simulink model "plantmodelwithcontroller"  (R2020a)
settings: Solver=VariableStepAuto  StartTime=0.0  StopTime=100  RelTol=1e-3
undefined symbols (not defined in the file): Ax, Ay, Az, b, d, g, I, Ixx, Iyy, Izz, Jr, m
libraries: simulink x4
settings Model: Creator=Muni Kumar  LastModifiedBy=Muni Kumar

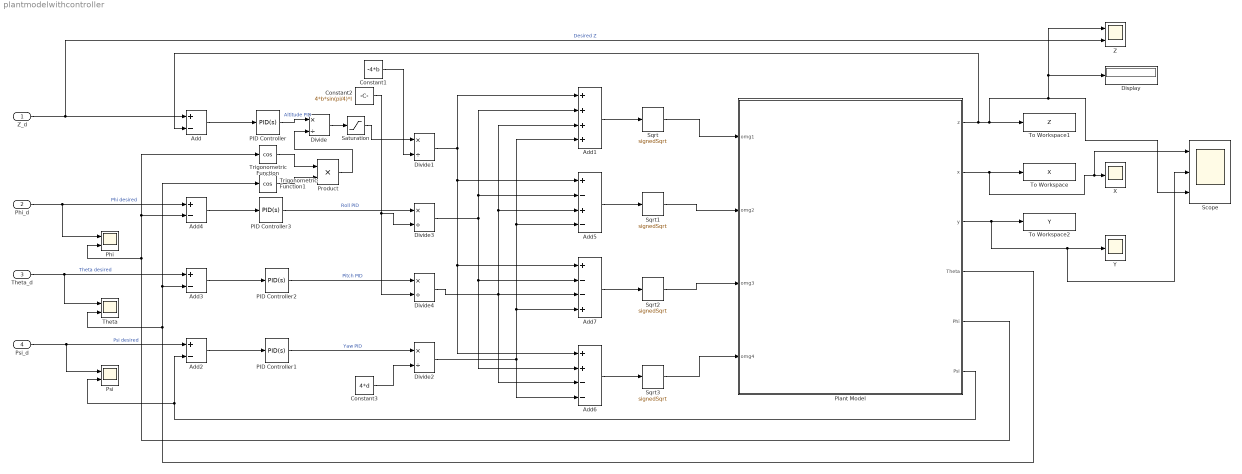
== system plantmodelwithcontroller ==
  Z_d : Inport
  Phi_d : Inport  Port=2
  Theta_d : Inport  Port=3
  Psi_d : Inport  Port=4
  Add{,2..4} (4 alike) : Sum  Inputs=+-
  Add1 : Sum  Inputs=++++
  Add5 : Sum  Inputs=+-+-
  Add6 : Sum  Inputs=++--
  Add7 : Sum  Inputs=+--+
  Constant1 : Constant  Value=-4*b
  Constant2 : Constant  Value=4*b*sin(pi/4)*I
  Constant3 : Constant  Value=4*d
  Display : Display
      settings: Decimation=2
  Divide{,1..4} (5 alike) : Product  Inputs=*/
  PID Controller : simulink/Continuous/PID Controller  Controller=PID  Form=Parallel  TimeDomain=Continuous-time  UseExternalTs=off  SampleTime=-1  IntegratorMethod=Forward Euler  FilterMethod=Forward Euler  ControllerParametersSource=internal  P=4  I=0  D=0  UseFilter=on  N=100  TunerSelectOption=Transfer Function Based (PID Tuner App)  InitialConditionSource=internal  InitialConditionForIntegrator=0  InitialConditionForFilter=0  DifferentiatorICPrevScaledInput=0  ExternalReset=none  TrackingMode=off  Kt=1  LimitOutput=off  UpperSaturationLimit=inf  LowerSaturationLimit=-inf  LinearizeAsGain=on  AntiWindupMode=none  Kb=1  POutMin=[]  POutMax=[]  IOutMin=[]  IOutMax=[]  DOutMin=[]  DOutMax=[]  NOutMin=[]  NOutMax=[]  SumOutMin=[]  SumOutMax=[]  SaturationOutMin=[]  SaturationOutMax=[]  PParamMin=[]  PParamMax=[]  IParamMin=[]  IParamMax=[]  DParamMin=[]  DParamMax=[]  NParamMin=[]  NParamMax=[]  KbParamMin=[]  KbParamMax=[]  KtParamMin=[]  KtParamMax=[]  KbOutMin=[]  KbOutMax=[]  KtOutMin=[]  KtOutMax=[]  IntegratorOutMin=[]  IntegratorOutMax=[]  FilterOutMin=[]  FilterOutMax=[]  SumI1OutMin=[]  SumI1OutMax=[]  SumI2OutMin=[]  SumI2OutMax=[]  SumI3OutMin=[]  SumI3OutMax=[]  SumI4OutMin=[]  SumI4OutMax=[]  SumDOutMin=[]  SumDOutMax=[]  DifferentiatorOutMin=[]  DifferentiatorOutMax=[]  FilterDiffOutCoefMin=[]  FilterDiffOutCoefMax=[]  ReciprocalOutMin=[]  ReciprocalOutMax=[]  SumDenOutMin=[]  SumDenOutMax=[]  SumNumOutMin=[]  SumNumOutMax=[]  DivideOutMin=[]  DivideOutMax=[]  UdiffTsProdOutMin=[]  UdiffTsProdOutMax=[]  NTsProdOutMin=[]  NTsProdOutMax=[]  UintegralTsProdOutMin=[]  UintegralTsProdOutMax=[]  UngainTsProdOutMin=[]  UngainTsProdOutMax=[]  IntegratorContinuousStateAttributes=''  IntegratorStateMustResolveToSignalObject=off  IntegratorRTWStateStorageClass=Auto  FilterContinuousStateAttributes=''  FilterStateMustResolveToSignalObject=off  FilterRTWStateStorageClass=Auto  ParallelPVariant=InternalParameters  IdealPVariant=Disabled  IVariant=InternalParameters  DVariant=InternalParameters  IntegratorVariant=Continuous  SatVariant=Disabled  AWVariant=Passthrough  PCopyVariant=Disabled  TRVariant=Disabled  FdbkBlocksVariant=Forward  IdealPFdbkVariant=Disabled  SatFdbkVariant=Disabled  DerivativeFilterVariant=ContFilter  NVariant=InternalParameters  NCopyVariant=Disabled  FilterICVariant=InternalICsFilter  IntegratorICVariant=InternalICs  ExternalResetVariant=Disabled  TRSumVariant=Passthrough  SumFdbkVariant=Disabled  SumVariant=Sum_PID  TsampFilterVariant=InternalTs  TsampNgainVariant=Passthrough  TsampIntegralVariant=Passthrough
  PID Controller1 : simulink/Continuous/PID Controller  Controller=PID  Form=Parallel  TimeDomain=Continuous-time  UseExternalTs=off  SampleTime=-1  IntegratorMethod=Forward Euler  FilterMethod=Forward Euler  ControllerParametersSource=internal  P=0.01  I=0.0002  D=0.03  UseFilter=on  N=100  TunerSelectOption=Transfer Function Based (PID Tuner App)  InitialConditionSource=internal  InitialConditionForIntegrator=0  InitialConditionForFilter=0  DifferentiatorICPrevScaledInput=0  ExternalReset=none  TrackingMode=off  Kt=1  LimitOutput=off  UpperSaturationLimit=inf  LowerSaturationLimit=-inf  LinearizeAsGain=on  AntiWindupMode=none  Kb=1  POutMin=[]  POutMax=[]  IOutMin=[]  IOutMax=[]  DOutMin=[]  DOutMax=[]  NOutMin=[]  NOutMax=[]  SumOutMin=[]  SumOutMax=[]  SaturationOutMin=[]  SaturationOutMax=[]  PParamMin=[]  PParamMax=[]  IParamMin=[]  IParamMax=[]  DParamMin=[]  DParamMax=[]  NParamMin=[]  NParamMax=[]  KbParamMin=[]  KbParamMax=[]  KtParamMin=[]  KtParamMax=[]  KbOutMin=[]  KbOutMax=[]  KtOutMin=[]  KtOutMax=[]  IntegratorOutMin=[]  IntegratorOutMax=[]  FilterOutMin=[]  FilterOutMax=[]  SumI1OutMin=[]  SumI1OutMax=[]  SumI2OutMin=[]  SumI2OutMax=[]  SumI3OutMin=[]  SumI3OutMax=[]  SumI4OutMin=[]  SumI4OutMax=[]  SumDOutMin=[]  SumDOutMax=[]  DifferentiatorOutMin=[]  DifferentiatorOutMax=[]  FilterDiffOutCoefMin=[]  FilterDiffOutCoefMax=[]  ReciprocalOutMin=[]  ReciprocalOutMax=[]  SumDenOutMin=[]  SumDenOutMax=[]  SumNumOutMin=[]  SumNumOutMax=[]  DivideOutMin=[]  DivideOutMax=[]  UdiffTsProdOutMin=[]  UdiffTsProdOutMax=[]  NTsProdOutMin=[]  NTsProdOutMax=[]  UintegralTsProdOutMin=[]  UintegralTsProdOutMax=[]  UngainTsProdOutMin=[]  UngainTsProdOutMax=[]  IntegratorContinuousStateAttributes=''  IntegratorStateMustResolveToSignalObject=off  IntegratorRTWStateStorageClass=Auto  FilterContinuousStateAttributes=''  FilterStateMustResolveToSignalObject=off  FilterRTWStateStorageClass=Auto  ParallelPVariant=InternalParameters  IdealPVariant=Disabled  IVariant=InternalParameters  DVariant=InternalParameters  IntegratorVariant=Continuous  SatVariant=Disabled  AWVariant=Passthrough  PCopyVariant=Disabled  TRVariant=Disabled  FdbkBlocksVariant=Forward  IdealPFdbkVariant=Disabled  SatFdbkVariant=Disabled  DerivativeFilterVariant=ContFilter  NVariant=InternalParameters  NCopyVariant=Disabled  FilterICVariant=InternalICsFilter  IntegratorICVariant=InternalICs  ExternalResetVariant=Disabled  TRSumVariant=Passthrough  SumFdbkVariant=Disabled  SumVariant=Sum_PID  TsampFilterVariant=InternalTs  TsampNgainVariant=Passthrough  TsampIntegralVariant=Passthrough
  PID Controller2 : simulink/Continuous/PID Controller  Controller=PID  Form=Parallel  TimeDomain=Continuous-time  UseExternalTs=off  SampleTime=-1  IntegratorMethod=Forward Euler  FilterMethod=Forward Euler  ControllerParametersSource=internal  P=0.006  I=0.000009  D=0.013  UseFilter=on  N=100  TunerSelectOption=Transfer Function Based (PID Tuner App)  InitialConditionSource=internal  InitialConditionForIntegrator=0  InitialConditionForFilter=0  DifferentiatorICPrevScaledInput=0  ExternalReset=none  TrackingMode=off  Kt=1  LimitOutput=off  UpperSaturationLimit=inf  LowerSaturationLimit=-inf  LinearizeAsGain=on  AntiWindupMode=none  Kb=1  POutMin=[]  POutMax=[]  IOutMin=[]  IOutMax=[]  DOutMin=[]  DOutMax=[]  NOutMin=[]  NOutMax=[]  SumOutMin=[]  SumOutMax=[]  SaturationOutMin=[]  SaturationOutMax=[]  PParamMin=[]  PParamMax=[]  IParamMin=[]  IParamMax=[]  DParamMin=[]  DParamMax=[]  NParamMin=[]  NParamMax=[]  KbParamMin=[]  KbParamMax=[]  KtParamMin=[]  KtParamMax=[]  KbOutMin=[]  KbOutMax=[]  KtOutMin=[]  KtOutMax=[]  IntegratorOutMin=[]  IntegratorOutMax=[]  FilterOutMin=[]  FilterOutMax=[]  SumI1OutMin=[]  SumI1OutMax=[]  SumI2OutMin=[]  SumI2OutMax=[]  SumI3OutMin=[]  SumI3OutMax=[]  SumI4OutMin=[]  SumI4OutMax=[]  SumDOutMin=[]  SumDOutMax=[]  DifferentiatorOutMin=[]  DifferentiatorOutMax=[]  FilterDiffOutCoefMin=[]  FilterDiffOutCoefMax=[]  ReciprocalOutMin=[]  ReciprocalOutMax=[]  SumDenOutMin=[]  SumDenOutMax=[]  SumNumOutMin=[]  SumNumOutMax=[]  DivideOutMin=[]  DivideOutMax=[]  UdiffTsProdOutMin=[]  UdiffTsProdOutMax=[]  NTsProdOutMin=[]  NTsProdOutMax=[]  UintegralTsProdOutMin=[]  UintegralTsProdOutMax=[]  UngainTsProdOutMin=[]  UngainTsProdOutMax=[]  IntegratorContinuousStateAttributes=''  IntegratorStateMustResolveToSignalObject=off  IntegratorRTWStateStorageClass=Auto  FilterContinuousStateAttributes=''  FilterStateMustResolveToSignalObject=off  FilterRTWStateStorageClass=Auto  ParallelPVariant=InternalParameters  IdealPVariant=Disabled  IVariant=InternalParameters  DVariant=InternalParameters  IntegratorVariant=Continuous  SatVariant=Disabled  AWVariant=Passthrough  PCopyVariant=Disabled  TRVariant=Disabled  FdbkBlocksVariant=Forward  IdealPFdbkVariant=Disabled  SatFdbkVariant=Disabled  DerivativeFilterVariant=ContFilter  NVariant=InternalParameters  NCopyVariant=Disabled  FilterICVariant=InternalICsFilter  IntegratorICVariant=InternalICs  ExternalResetVariant=Disabled  TRSumVariant=Passthrough  SumFdbkVariant=Disabled  SumVariant=Sum_PID  TsampFilterVariant=InternalTs  TsampNgainVariant=Passthrough  TsampIntegralVariant=Passthrough
  PID Controller3 : simulink/Continuous/PID Controller  Controller=PID  Form=Parallel  TimeDomain=Continuous-time  UseExternalTs=off  SampleTime=-1  IntegratorMethod=Forward Euler  FilterMethod=Forward Euler  ControllerParametersSource=internal  P=0.006  I=0.000009  D=0.013  UseFilter=on  N=100  TunerSelectOption=Transfer Function Based (PID Tuner App)  InitialConditionSource=internal  InitialConditionForIntegrator=0  InitialConditionForFilter=0  DifferentiatorICPrevScaledInput=0  ExternalReset=none  TrackingMode=off  Kt=1  LimitOutput=off  UpperSaturationLimit=inf  LowerSaturationLimit=-inf  LinearizeAsGain=on  AntiWindupMode=none  Kb=1  POutMin=[]  POutMax=[]  IOutMin=[]  IOutMax=[]  DOutMin=[]  DOutMax=[]  NOutMin=[]  NOutMax=[]  SumOutMin=[]  SumOutMax=[]  SaturationOutMin=[]  SaturationOutMax=[]  PParamMin=[]  PParamMax=[]  IParamMin=[]  IParamMax=[]  DParamMin=[]  DParamMax=[]  NParamMin=[]  NParamMax=[]  KbParamMin=[]  KbParamMax=[]  KtParamMin=[]  KtParamMax=[]  KbOutMin=[]  KbOutMax=[]  KtOutMin=[]  KtOutMax=[]  IntegratorOutMin=[]  IntegratorOutMax=[]  FilterOutMin=[]  FilterOutMax=[]  SumI1OutMin=[]  SumI1OutMax=[]  SumI2OutMin=[]  SumI2OutMax=[]  SumI3OutMin=[]  SumI3OutMax=[]  SumI4OutMin=[]  SumI4OutMax=[]  SumDOutMin=[]  SumDOutMax=[]  DifferentiatorOutMin=[]  DifferentiatorOutMax=[]  FilterDiffOutCoefMin=[]  FilterDiffOutCoefMax=[]  ReciprocalOutMin=[]  ReciprocalOutMax=[]  SumDenOutMin=[]  SumDenOutMax=[]  SumNumOutMin=[]  SumNumOutMax=[]  DivideOutMin=[]  DivideOutMax=[]  UdiffTsProdOutMin=[]  UdiffTsProdOutMax=[]  NTsProdOutMin=[]  NTsProdOutMax=[]  UintegralTsProdOutMin=[]  UintegralTsProdOutMax=[]  UngainTsProdOutMin=[]  UngainTsProdOutMax=[]  IntegratorContinuousStateAttributes=''  IntegratorStateMustResolveToSignalObject=off  IntegratorRTWStateStorageClass=Auto  FilterContinuousStateAttributes=''  FilterStateMustResolveToSignalObject=off  FilterRTWStateStorageClass=Auto  ParallelPVariant=InternalParameters  IdealPVariant=Disabled  IVariant=InternalParameters  DVariant=InternalParameters  IntegratorVariant=Continuous  SatVariant=Disabled  AWVariant=Passthrough  PCopyVariant=Disabled  TRVariant=Disabled  FdbkBlocksVariant=Forward  IdealPFdbkVariant=Disabled  SatFdbkVariant=Disabled  DerivativeFilterVariant=ContFilter  NVariant=InternalParameters  NCopyVariant=Disabled  FilterICVariant=InternalICsFilter  IntegratorICVariant=InternalICs  ExternalResetVariant=Disabled  TRSumVariant=Passthrough  SumFdbkVariant=Disabled  SumVariant=Sum_PID  TsampFilterVariant=InternalTs  TsampNgainVariant=Passthrough  TsampIntegralVariant=Passthrough
  Phi : Scope  NumInputPorts=2
  Plant Model : Subsystem
  Product : Product
  Psi : Scope  NumInputPorts=2
  Saturation : Saturate
  Scope : Scope  NumInputPorts=3
  Sqrt{,1..3} (4 alike) : Sqrt  Operator=signedSqrt  SaturateOnIntegerOverflow=on
  Theta : Scope  NumInputPorts=2
  To Workspace : ToWorkspace  VariableName=X  SaveFormat=Timeseries  SampleTime=-1
  To Workspace1 : ToWorkspace  VariableName=Z  SaveFormat=Timeseries  SampleTime=-1
  To Workspace2 : ToWorkspace  VariableName=Y  SaveFormat=Timeseries  SampleTime=-1
  Trigonometric Function : Trigonometry  Operator=cos
  Trigonometric Function1 : Trigonometry  Operator=cos
  X : Scope
  Y : Scope
  Z : Scope  NumInputPorts=2
  wires:
  Psi_d/1 -> Psi/1, Add2/1  "Psi desired"
  Divide4/1 -> Add6/3, Add5/3, Add1/3, Add7/3
  Add5/1 -> Sqrt1/1
  Theta_d/1 -> Theta/1, Add3/1  "Theta desired"
  Add2/1 -> PID Controller1/1
  Add6/1 -> Sqrt3/1
  Divide3/1 -> Add7/2, Add6/2, Add5/2, Add1/2
  Constant3/1 -> Divide2/2
  Constant1/1 -> Divide1/2
  Add1/1 -> Sqrt/1
  Z_d/1 -> Z/2, Add/1  "Desired Z"
  Add/1 -> PID Controller/1
  PID Controller2/1 -> Divide4/1  "Pitch PID"
  Constant2/1 -> Divide3/2, Divide4/2
  Phi_d/1 -> Phi/1, Add4/1  "Phi desired"
  PID Controller1/1 -> Divide2/1  "Yaw PID"
  Divide2/1 -> Add6/4, Add7/4, Add5/4, Add1/4
  Trigonometric Function1/1 -> Product/2
  Divide1/1 -> Add5/1, Add7/1, Add6/1, Add1/1
  Add7/1 -> Sqrt2/1
  Divide/1 -> Saturation/1
  Add4/1 -> PID Controller3/1
  PID Controller/1 -> Divide/1  "Altitude PID"
  PID Controller3/1 -> Divide3/1  "Roll PID"
  Trigonometric Function/1 -> Product/1
  Add3/1 -> PID Controller2/1
  Plant Model/1(z) -> Add/2, Display/1, Z/1, Scope/3, To Workspace1/1
  Plant Model/3(y) -> Scope/2, Y/1, To Workspace2/1
  Plant Model/4(Theta) -> Theta/2, Add3/2, Trigonometric Function1/1
  Plant Model/5(Phi) -> Phi/2, Add4/2, Trigonometric Function/1
  Sqrt/1 -> Plant Model/1(omg1)
  Sqrt1/1 -> Plant Model/2(omg2)
  Sqrt2/1 -> Plant Model/3(omg3)
  Sqrt3/1 -> Plant Model/4(omg4)
  Product/1 -> Divide/2
  Plant Model/6(Psi) -> Psi/2, Add2/2
  Plant Model/2(x) -> X/1, Scope/1, To Workspace/1
  Saturation/1 -> Divide1/1

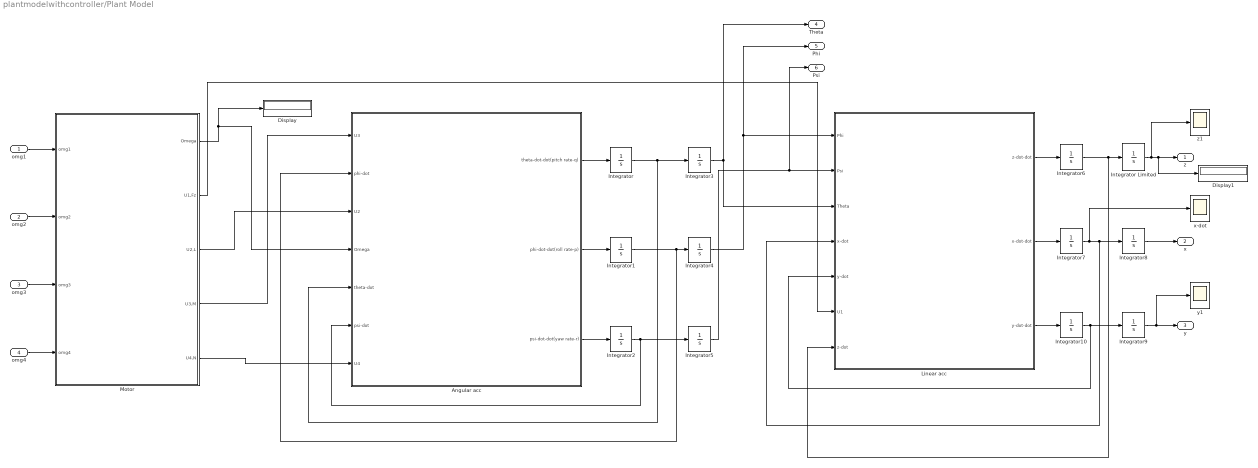
== system plantmodelwithcontroller/Plant Model ==
  omg1 : Inport
  omg2 : Inport  Port=2
  omg3 : Inport  Port=3
  omg4 : Inport  Port=4
  Angular acc : Subsystem
  Display : Display
      settings: Decimation=2
  Display1 : Display
  Integrator{,1..2,6..10} (8 alike) : Integrator
  Integrator Limited : Integrator  LimitOutput=on  UpperSaturationLimit=0  IgnoreLimit=on
  Integrator3 : Integrator  WrapState=on
  Integrator4 : Integrator  WrapState=on
  Integrator5 : Integrator  WrapState=on
  Linear acc : Subsystem
  Motor : Subsystem
  x-dot : Scope
  y1 : Scope
  z1 : Scope
  z : Outport
  x : Outport  Port=2
  y : Outport  Port=3
  Theta : Outport  Port=4
  Phi : Outport  Port=5
  Psi : Outport  Port=6
  wires:
  Motor/2(U1,Fz) -> Linear acc/6(U1)
  omg3/1 -> Motor/3(omg3)
  Integrator6/1 -> Integrator Limited/1, Linear acc/7(z-dot)
  Angular acc/2(phi-dot-dot(roll rate-p)) -> Integrator1/1
  Integrator7/1 -> x-dot/1, Linear acc/4(x-dot), Integrator8/1
  Integrator3/1 -> Theta/1, Linear acc/3(Theta)
  Motor/5(U4,N) -> Angular acc/7(U4)
  Angular acc/3(psi-dot-dot(yaw rate-r)) -> Integrator2/1
  Integrator10/1 -> Integrator9/1, Linear acc/5(y-dot)
  omg1/1 -> Motor/1(omg1)
  Angular acc/1(theta-dot-dot(pitch rate-q)) -> Integrator/1
  Integrator5/1 -> Psi/1, Linear acc/2(Psi)
  Linear acc/2(x-dot-dot) -> Integrator7/1
  Motor/3(U2,L) -> Angular acc/3(U2)
  Integrator4/1 -> Phi/1, Linear acc/1(Phi)
  Integrator/1 -> Angular acc/5(theta-dot), Integrator3/1
  Integrator9/1 -> y/1, y1/1
  Linear acc/3(y-dot-dot) -> Integrator10/1
  omg4/1 -> Motor/4(omg4)
  Integrator Limited/1 -> z1/1, z/1, Display1/1
  Integrator2/1 -> Angular acc/6(psi-dot), Integrator5/1
  Linear acc/1(z-dot-dot) -> Integrator6/1
  Motor/1(Omega) -> Display/1, Angular acc/4(Omega)
  Integrator8/1 -> x/1
  Motor/4(U3,M) -> Angular acc/1(U3)
  Integrator1/1 -> Angular acc/2(phi-dot), Integrator4/1
  omg2/1 -> Motor/2(omg2)

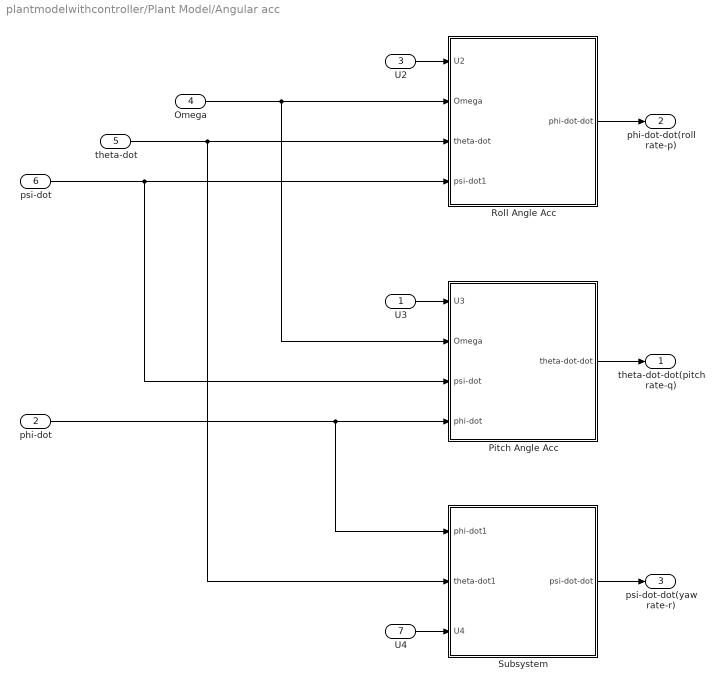
== system plantmodelwithcontroller/Plant Model/Angular acc ==
  U3 : Inport
  phi-dot : Inport  Port=2
  U2 : Inport  Port=3
  Omega : Inport  Port=4
  theta-dot : Inport  Port=5
  psi-dot : Inport  Port=6
  U4 : Inport  Port=7
  Pitch Angle Acc : Subsystem
  Roll Angle Acc : Subsystem
  Subsystem : Subsystem
  theta-dot-dot(pitch rate-q) : Outport
  phi-dot-dot(roll rate-p) : Outport  Port=2
  psi-dot-dot(yaw rate-r) : Outport  Port=3
  wires:
  phi-dot/1 -> Subsystem/1(phi-dot1), Pitch Angle Acc/4(phi-dot)
  U2/1 -> Roll Angle Acc/1(U2)
  Roll Angle Acc/1(phi-dot-dot) -> phi-dot-dot(roll rate-p)/1
  U4/1 -> Subsystem/3(U4)
  theta-dot/1 -> Subsystem/2(theta-dot1), Roll Angle Acc/3(theta-dot)
  Subsystem/1(psi-dot-dot) -> psi-dot-dot(yaw rate-r)/1
  psi-dot/1 -> Pitch Angle Acc/3(psi-dot), Roll Angle Acc/4(psi-dot1)
  Pitch Angle Acc/1(theta-dot-dot) -> theta-dot-dot(pitch rate-q)/1
  U3/1 -> Pitch Angle Acc/1(U3)
  Omega/1 -> Pitch Angle Acc/2(Omega), Roll Angle Acc/2(Omega)

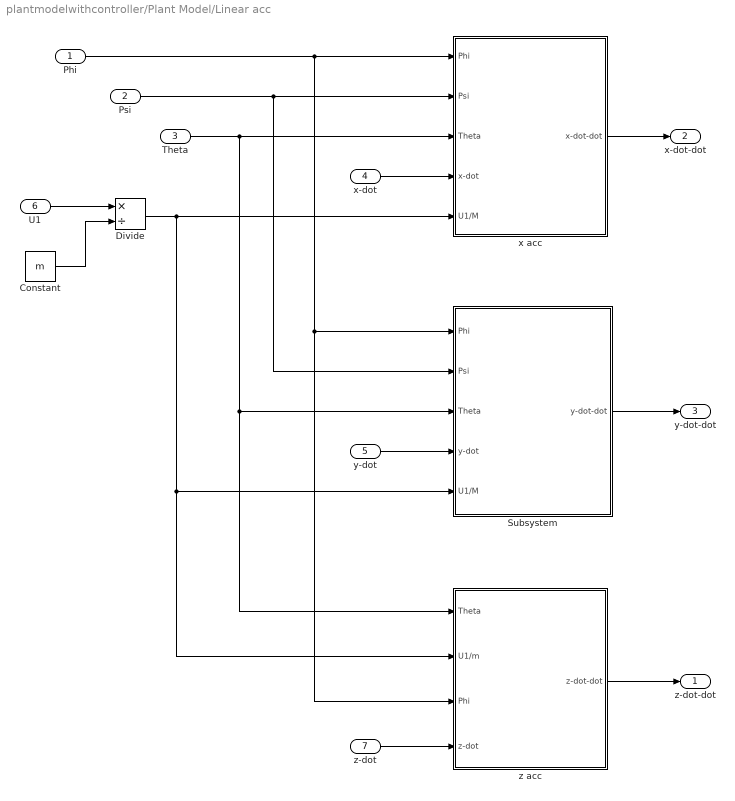
== system plantmodelwithcontroller/Plant Model/Linear acc ==
  Phi : Inport
  Psi : Inport  Port=2
  Theta : Inport  Port=3
  x-dot : Inport  Port=4
  y-dot : Inport  Port=5
  U1 : Inport  Port=6
  z-dot : Inport  Port=7
  Constant : Constant  Value=m
  Divide : Product  Inputs=*/
  Subsystem : Subsystem
  x acc : Subsystem
  z acc : Subsystem
  z-dot-dot : Outport
  x-dot-dot : Outport  Port=2
  y-dot-dot : Outport  Port=3
  wires:
  Theta/1 -> x acc/3(Theta), Subsystem/3(Theta), z acc/1(Theta)
  Phi/1 -> Subsystem/1(Phi), z acc/3(Phi), x acc/1(Phi)
  Divide/1 -> Subsystem/5(U1/M), z acc/2(U1/m), x acc/5(U1/M)
  y-dot/1 -> Subsystem/4(y-dot)
  Constant/1 -> Divide/2
  Psi/1 -> Subsystem/2(Psi), x acc/2(Psi)
  z-dot/1 -> z acc/4(z-dot)
  U1/1 -> Divide/1
  x-dot/1 -> x acc/4(x-dot)
  x acc/1(x-dot-dot) -> x-dot-dot/1
  z acc/1(z-dot-dot) -> z-dot-dot/1
  Subsystem/1(y-dot-dot) -> y-dot-dot/1

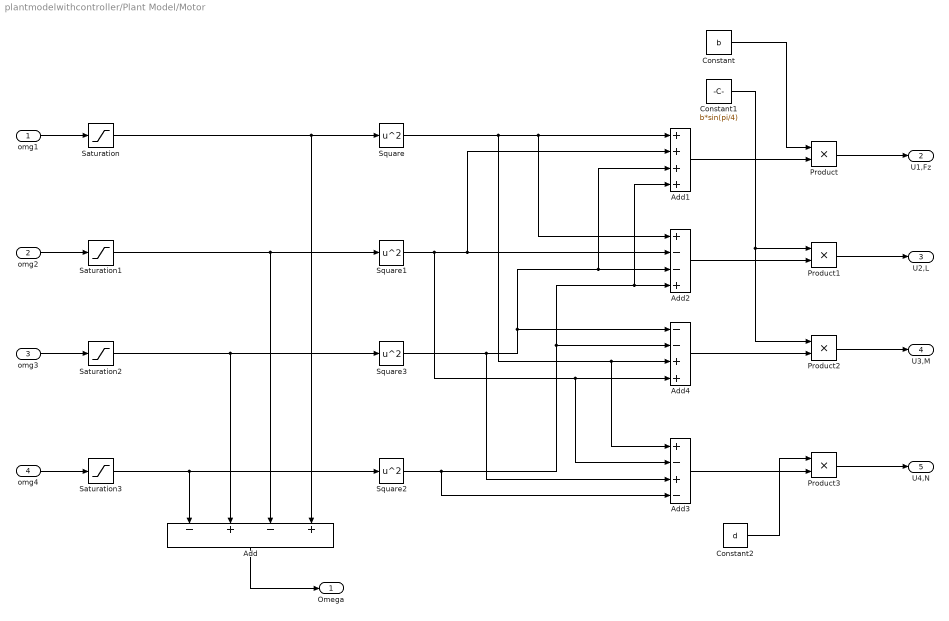
== system plantmodelwithcontroller/Plant Model/Motor ==
  omg1 : Inport
  omg2 : Inport  Port=2
  omg3 : Inport  Port=3
  omg4 : Inport  Port=4
  Add : Sum  Inputs=-+-+
  Add1 : Sum  Inputs=++++
  Add2 : Sum  Inputs=+--+
  Add3 : Sum  Inputs=+-+-
  Add4 : Sum  Inputs=--++
  Constant : Constant  Value=b
  Constant1 : Constant  Value=b*sin(pi/4)
  Constant2 : Constant  Value=d
  Product{,1..3} (4 alike) : Product
  Saturation{,1..3} (4 alike) : Saturate  UpperLimit=inf  LowerLimit=0
  Square{,1..3} (4 alike) : Math  Operator=square  SaturateOnIntegerOverflow=on
  Omega : Outport
  U1,Fz : Outport  Port=2
  U2,L : Outport  Port=3
  U3,M : Outport  Port=4
  U4,N : Outport  Port=5
  wires:
  Product3/1 -> U4,N/1
  omg1/1 -> Saturation/1
  omg2/1 -> Saturation1/1
  Add/1 -> Omega/1
  omg3/1 -> Saturation2/1
  Product2/1 -> U3,M/1
  Saturation/1 -> Add/4, Square/1
  Product1/1 -> U2,L/1
  Product/1 -> U1,Fz/1
  Add2/1 -> Product1/2
  Square3/1 -> Add3/3, Add4/1, Add1/3, Add2/3
  Square2/1 -> Add4/2, Add1/4, Add2/4, Add3/4
  Square/1 -> Add3/1, Add4/3, Add2/1, Add1/1
  Saturation3/1 -> Add/1, Square2/1
  Constant/1 -> Product/1
  Square1/1 -> Add3/2, Add4/4, Add1/2, Add2/2
  omg4/1 -> Saturation3/1
  Constant1/1 -> Product2/1, Product1/1
  Add4/1 -> Product2/2
  Add1/1 -> Product/2
  Add3/1 -> Product3/2
  Saturation2/1 -> Add/2, Square3/1
  Saturation1/1 -> Add/3, Square1/1
  Constant2/1 -> Product3/1

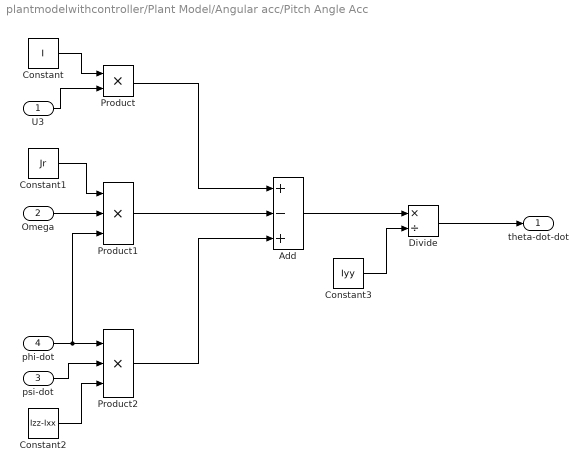
== system plantmodelwithcontroller/Plant Model/Angular acc/Pitch Angle Acc ==
  U3 : Inport
  Omega : Inport  Port=2
  psi-dot : Inport  Port=3
  phi-dot : Inport  Port=4
  Add : Sum  Inputs=+-+
  Constant : Constant  Value=I
  Constant1 : Constant  Value=Jr
  Constant2 : Constant  Value=Izz-Ixx
  Constant3 : Constant  Value=Iyy
  Divide : Product  Inputs=*/
  Product : Product
  Product1 : Product  Inputs=3
  Product2 : Product  Inputs=3
  theta-dot-dot : Outport
  wires:
  Divide/1 -> theta-dot-dot/1
  Product/1 -> Add/1
  phi-dot/1 -> Product1/3, Product2/1
  psi-dot/1 -> Product2/2
  Product1/1 -> Add/2
  Constant1/1 -> Product1/1
  U3/1 -> Product/2
  Constant/1 -> Product/1
  Constant3/1 -> Divide/2
  Constant2/1 -> Product2/3
  Omega/1 -> Product1/2
  Add/1 -> Divide/1
  Product2/1 -> Add/3

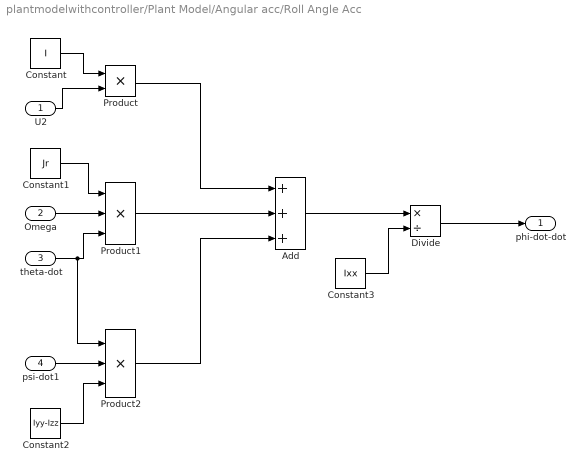
== system plantmodelwithcontroller/Plant Model/Angular acc/Roll Angle Acc ==
  U2 : Inport
  Omega : Inport  Port=2
  theta-dot : Inport  Port=3
  psi-dot1 : Inport  Port=4
  Add : Sum  Inputs=+++
  Constant : Constant  Value=I
  Constant1 : Constant  Value=Jr
  Constant2 : Constant  Value=Iyy-Izz
  Constant3 : Constant  Value=Ixx
  Divide : Product  Inputs=*/
  Product : Product
  Product1 : Product  Inputs=3
  Product2 : Product  Inputs=3
  phi-dot-dot : Outport
  wires:
  psi-dot1/1 -> Product2/2
  Product/1 -> Add/1
  Constant/1 -> Product/1
  theta-dot/1 -> Product2/1, Product1/3
  Product1/1 -> Add/2
  Constant3/1 -> Divide/2
  Add/1 -> Divide/1
  Constant2/1 -> Product2/3
  Product2/1 -> Add/3
  U2/1 -> Product/2
  Omega/1 -> Product1/2
  Constant1/1 -> Product1/1
  Divide/1 -> phi-dot-dot/1

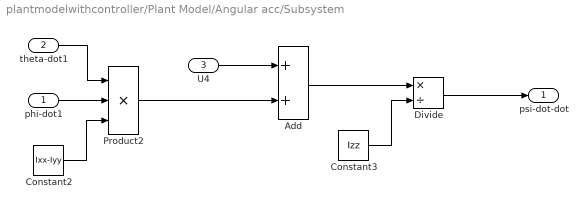
== system plantmodelwithcontroller/Plant Model/Angular acc/Subsystem ==
  phi-dot1 : Inport
  theta-dot1 : Inport  Port=2
  U4 : Inport  Port=3
  Add : Sum
  Constant2 : Constant  Value=Ixx-Iyy
  Constant3 : Constant  Value=Izz
  Divide : Product  Inputs=*/
  Product2 : Product  Inputs=3
  psi-dot-dot : Outport
  wires:
  Constant2/1 -> Product2/3
  phi-dot1/1 -> Product2/2
  Product2/1 -> Add/2
  theta-dot1/1 -> Product2/1
  Constant3/1 -> Divide/2
  Add/1 -> Divide/1
  U4/1 -> Add/1
  Divide/1 -> psi-dot-dot/1

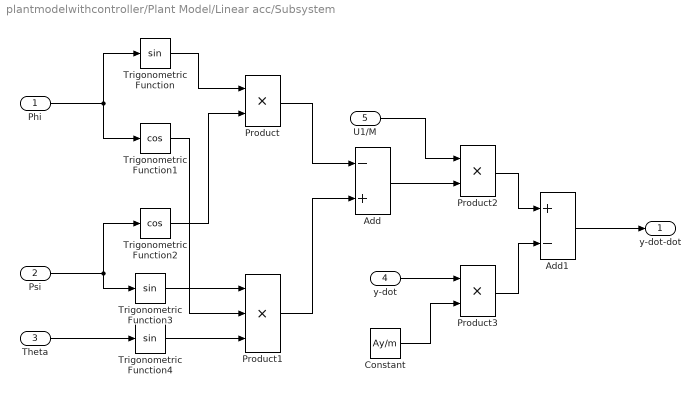
== system plantmodelwithcontroller/Plant Model/Linear acc/Subsystem ==
  Phi : Inport
  Psi : Inport  Port=2
  Theta : Inport  Port=3
  y-dot : Inport  Port=4
  U1/M : Inport  Port=5
  Add : Sum  Inputs=-+
  Add1 : Sum  Inputs=+-
  Constant : Constant  Value=Ay/m
  Product : Product
  Product1 : Product  Inputs=3
  Product2 : Product
  Product3 : Product
  Trigonometric Function : Trigonometry
  Trigonometric Function1 : Trigonometry  Operator=cos
  Trigonometric Function2 : Trigonometry  Operator=cos
  Trigonometric Function3 : Trigonometry
  Trigonometric Function4 : Trigonometry
  y-dot-dot : Outport
  wires:
  Phi/1 -> Trigonometric Function1/1, Trigonometric Function/1
  Theta/1 -> Trigonometric Function4/1
  Trigonometric Function1/1 -> Product1/2
  Add1/1 -> y-dot-dot/1
  Psi/1 -> Trigonometric Function3/1, Trigonometric Function2/1
  Trigonometric Function4/1 -> Product1/3
  y-dot/1 -> Product3/1
  Product2/1 -> Add1/1
  U1/M/1 -> Product2/1
  Product1/1 -> Add/2
  Add/1 -> Product2/2
  Constant/1 -> Product3/2
  Product/1 -> Add/1
  Trigonometric Function3/1 -> Product1/1
  Product3/1 -> Add1/2
  Trigonometric Function/1 -> Product/1
  Trigonometric Function2/1 -> Product/2

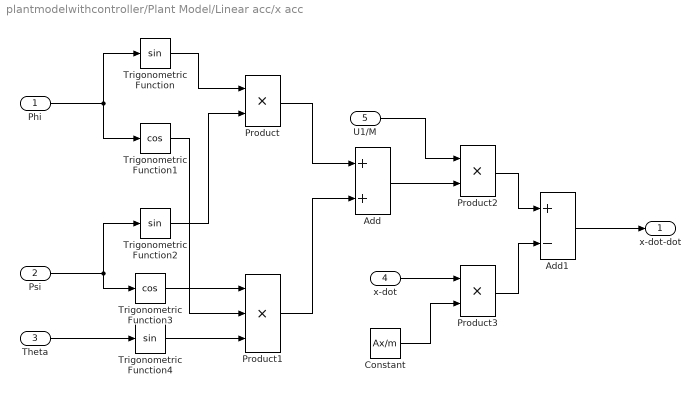
== system plantmodelwithcontroller/Plant Model/Linear acc/x acc ==
  Phi : Inport
  Psi : Inport  Port=2
  Theta : Inport  Port=3
  x-dot : Inport  Port=4
  U1/M : Inport  Port=5
  Add : Sum
  Add1 : Sum  Inputs=+-
  Constant : Constant  Value=Ax/m
  Product : Product
  Product1 : Product  Inputs=3
  Product2 : Product
  Product3 : Product
  Trigonometric Function : Trigonometry
  Trigonometric Function1 : Trigonometry  Operator=cos
  Trigonometric Function2 : Trigonometry
  Trigonometric Function3 : Trigonometry  Operator=cos
  Trigonometric Function4 : Trigonometry
  x-dot-dot : Outport
  wires:
  Phi/1 -> Trigonometric Function1/1, Trigonometric Function/1
  x-dot/1 -> Product3/1
  Product3/1 -> Add1/2
  U1/M/1 -> Product2/1
  Psi/1 -> Trigonometric Function3/1, Trigonometric Function2/1
  Trigonometric Function3/1 -> Product1/1
  Theta/1 -> Trigonometric Function4/1
  Add/1 -> Product2/2
  Trigonometric Function1/1 -> Product1/2
  Trigonometric Function2/1 -> Product/2
  Product1/1 -> Add/2
  Product2/1 -> Add1/1
  Trigonometric Function/1 -> Product/1
  Trigonometric Function4/1 -> Product1/3
  Product/1 -> Add/1
  Constant/1 -> Product3/2
  Add1/1 -> x-dot-dot/1

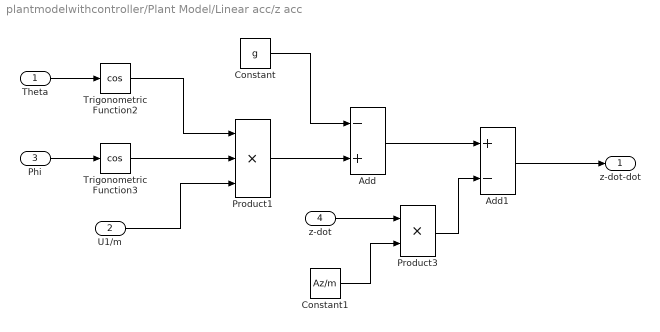
== system plantmodelwithcontroller/Plant Model/Linear acc/z acc ==
  Theta : Inport
  U1/m : Inport  Port=2
  Phi : Inport  Port=3
  z-dot : Inport  Port=4
  Add : Sum  Inputs=-+
  Add1 : Sum  Inputs=+-
  Constant : Constant  Value=g
  Constant1 : Constant  Value=Az/m
  Product1 : Product  Inputs=3
  Product3 : Product
  Trigonometric Function2 : Trigonometry  Operator=cos
  Trigonometric Function3 : Trigonometry  Operator=cos
  z-dot-dot : Outport
  wires:
  Phi/1 -> Trigonometric Function3/1
  Product3/1 -> Add1/2
  U1/m/1 -> Product1/3
  Theta/1 -> Trigonometric Function2/1
  Add/1 -> Add1/1
  Product1/1 -> Add/2
  Add1/1 -> z-dot-dot/1
  Constant1/1 -> Product3/2
  z-dot/1 -> Product3/1
  Trigonometric Function3/1 -> Product1/2
  Constant/1 -> Add/1
  Trigonometric Function2/1 -> Product1/1
